simulink library "util_thruster_lib"  (R2014b)
settings: Solver=ode45  SolverMode=SingleTasking  StartTime=0.0  StopTime=10.0  RelTol=1e-3
undefined symbols (not defined in the file): cg
libraries: util_common_lib x5
settings Model: Creator=dviazzo  LastModifiedBy=mstewart

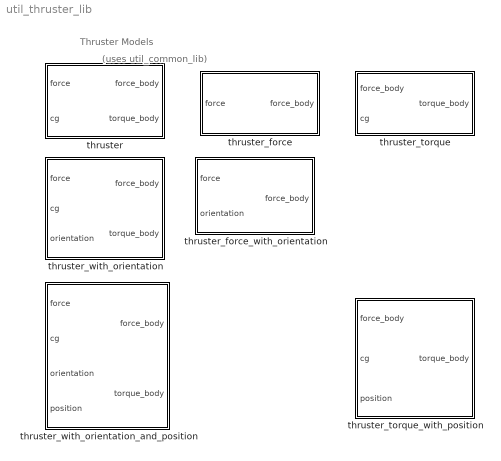
== system util_thruster_lib ==
  note: Thruster Models
  note: (uses util_common_lib)
  thruster : Subsystem  mask(Thruster){Thruster_Position=, Thruster_Orientation=}
      mask prompts: Thruster_Position "Enter thruster position in Body Frame"; Thruster_Orientation "Enter thruster orientation in Body Frame"
      mask Display:
      | color('blue')
      | text(0.05,0.02,'NASA',...
      |  	'HorizontalAlignment','Left',...
      | 	'VerticalAlignment','bottom')
  thruster_force : Subsystem  mask(Thruster){Thruster_Orientation=[]}
      mask prompts: Thruster_Orientation "Enter thruster orientation in Body Frame"
      mask Display:
      | color('blue')
      | text(0.05,0.02,'NASA',...
      |  	'HorizontalAlignment','Left',...
      | 	'VerticalAlignment','bottom')
  thruster_force_with_orientation : Subsystem  mask(Thruster){}
      mask help: Generic thruster model
      mask Display:
      | color('blue')
      | text(0.05,0.02,'NASA',...
      |  	'HorizontalAlignment','Left',...
      | 	'VerticalAlignment','bottom')
  thruster_torque : Subsystem  mask(Thruster){Thruster_Position=cg}
      mask prompts: Thruster_Position "Enter thruster position in Body Frame"
      mask Display:
      | color('blue')
      | text(0.05,0.02,'NASA',...
      |  	'HorizontalAlignment','Left',...
      | 	'VerticalAlignment','bottom')
  thruster_torque_with_position : Subsystem  mask(Thruster){}
      mask help: This is a general thruster model
      mask Display:
      | color('blue')
      | text(0.05,0.02,'NASA',...
      |  	'HorizontalAlignment','Left',...
      | 	'VerticalAlignment','bottom')
  thruster_with_orientation : Subsystem  mask(Thruster){Thruster_Position=[]}
      mask prompts: Thruster_Position "Enter thruster position in Body Frame"
      mask Display:
      | color('blue')
      | text(0.05,0.02,'NASA',...
      |  	'HorizontalAlignment','Left',...
      | 	'VerticalAlignment','bottom')
  thruster_with_orientation_and_position : Subsystem  mask(Thruster){}
      mask help: This is a general thruster model
      mask Display:
      | color('blue')
      | text(0.05,0.02,'NASA',...
      |  	'HorizontalAlignment','Left',...
      | 	'VerticalAlignment','bottom')

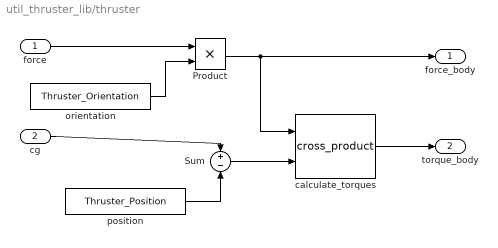
== system util_thruster_lib/thruster ==
  force : Inport
  cg : Inport  Port=2
  Product : Product  RndMeth=Zero
  Sum : Sum  Inputs=+-
  calculate_torques : util_common_lib/cross_product  SystemSampleTime=-1
  orientation : Constant  Value=Thruster_Orientation
  position : Constant  Value=Thruster_Position
  force_body : Outport
  torque_body : Outport  Port=2
  wires:
  Sum/1 -> calculate_torques/2
  cg/1 -> Sum/1
  force/1 -> Product/1
  orientation/1 -> Product/2
  Product/1 -> force_body/1, calculate_torques/1
  calculate_torques/1 -> torque_body/1
  position/1 -> Sum/2

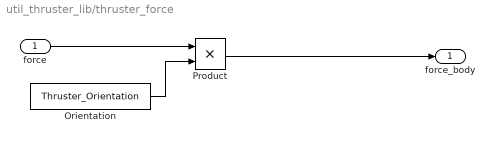
== system util_thruster_lib/thruster_force ==
  force : Inport
  Orientation : Constant  Value=Thruster_Orientation
  Product : Product  RndMeth=Zero
  force_body : Outport
  wires:
  Product/1 -> force_body/1
  Orientation/1 -> Product/2
  force/1 -> Product/1

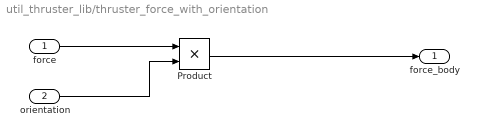
== system util_thruster_lib/thruster_force_with_orientation ==
  force : Inport
  orientation : Inport  Port=2
  Product : Product  RndMeth=Zero
  force_body : Outport
  wires:
  force/1 -> Product/1
  orientation/1 -> Product/2
  Product/1 -> force_body/1

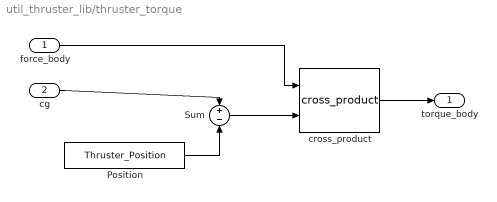
== system util_thruster_lib/thruster_torque ==
  force_body : Inport
  cg : Inport  Port=2
  Position : Constant  Value=Thruster_Position
  Sum : Sum  Inputs=+-
  cross_product : util_common_lib/cross_product  SystemSampleTime=-1
  torque_body : Outport
  wires:
  Position/1 -> Sum/2
  cross_product/1 -> torque_body/1
  cg/1 -> Sum/1
  Sum/1 -> cross_product/2
  force_body/1 -> cross_product/1

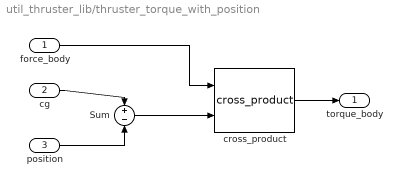
== system util_thruster_lib/thruster_torque_with_position ==
  force_body : Inport
  cg : Inport  Port=2
  position : Inport  Port=3
  Sum : Sum  Inputs=+-
  cross_product : util_common_lib/cross_product  SystemSampleTime=-1
  torque_body : Outport
  wires:
  position/1 -> Sum/2
  cross_product/1 -> torque_body/1
  cg/1 -> Sum/1
  Sum/1 -> cross_product/2
  force_body/1 -> cross_product/1

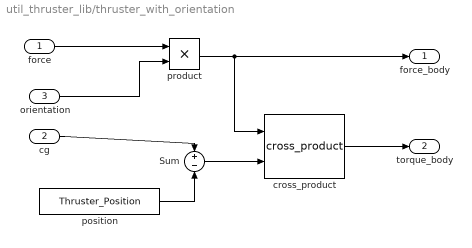
== system util_thruster_lib/thruster_with_orientation ==
  force : Inport
  cg : Inport  Port=2
  orientation : Inport  Port=3
  Sum : Sum  Inputs=+-
  cross_product : util_common_lib/cross_product  SystemSampleTime=-1
  position : Constant  Value=Thruster_Position
  product : Product  RndMeth=Zero
  force_body : Outport
  torque_body : Outport  Port=2
  wires:
  position/1 -> Sum/2
  cross_product/1 -> torque_body/1
  product/1 -> force_body/1, cross_product/1
  orientation/1 -> product/2
  force/1 -> product/1
  cg/1 -> Sum/1
  Sum/1 -> cross_product/2

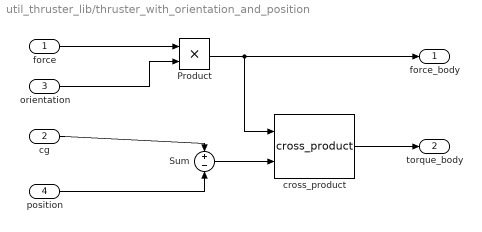
== system util_thruster_lib/thruster_with_orientation_and_position ==
  force : Inport
  cg : Inport  Port=2
  orientation : Inport  Port=3
  position : Inport  Port=4
  Product : Product  RndMeth=Zero
  Sum : Sum  Inputs=+-
  cross_product : util_common_lib/cross_product  SystemSampleTime=-1
  force_body : Outport
  torque_body : Outport  Port=2
  wires:
  Sum/1 -> cross_product/2
  cg/1 -> Sum/1
  force/1 -> Product/1
  orientation/1 -> Product/2
  Product/1 -> force_body/1, cross_product/1
  cross_product/1 -> torque_body/1
  position/1 -> Sum/2
